simulink model "ckt_notime"  (R2017b)
settings: Solver=VariableStepAuto  StartTime=0.0  StopTime=37790  MaxStep=1e-4  RelTol=1e-3
undefined symbols (not defined in the file or in its folder): sigbuilder_block, Ts_Power
libraries: powerlib x10, re_lib x1, powerlib_meascontrol x1
settings Model: Creator=VSS  LastModifiedBy=VSSDEEP

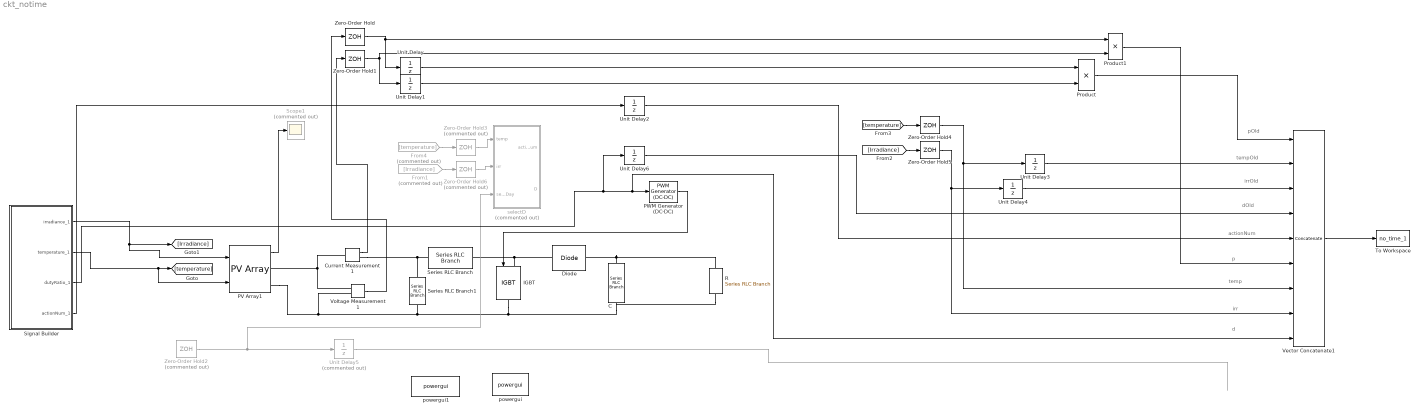
== system ckt_notime ==
  note: d
  note: irr
  note: temp
  note: p
  note: actionNum
  note: dOld
  note: tempOld
  note: irrOld
  note: pOld
  C : powerlib/Elements/Series RLC Branch  LConnTagsString=__new0  RConnTagsString=__new0  BranchType=C  Resistance=5e-3  Inductance=1e-3  SetiL0=off  InitialCurrent=0  Capacitance=330e-6  Setx0=off  InitialVoltage=0  Measurements=None
  Current Measurement1 : powerlib/Measurements/Current Measurement  PhasorSimulation=off  OutputType=Complex  PSBequivalent=0
  Diode : powerlib/Power Electronics/Diode  Ron=0.001  Lon=0  Vf=0.8  IC=0  UseSnubber=off  Rs=500  Cs=250e-9  Measurements=off
  From1 : From  Commented=on  GotoTag=Irradiance
  From4 : From  Commented=on  GotoTag=temperature
  IGBT : powerlib/Power Electronics/IGBT  Ron=0.001  Lon=0  Vf=0  Tf=1e-6  Tt=2e-6  IC=0  Rs=1e5  Cs=inf  Measurements=off
  PV Array1 : re_lib/Solar/PV Array  Npar=1  Nser=1  PlotType=one module @ 25 deg.C & specified irradiances  S_vec="[ 1000  500  100 ]"  Temp_C_vec="[ 45 25  ]"  ModuleName=User-defined  PlotWhenSelected=off  Pm=49.86  Ncell=36  Voc=21.24  Isc=3.05  Vm=18  Im=2.77  beta_Voc_pc=-0.36099  alpha_Isc_pc=0.102  beta_Voc=-0.076674  alpha_Isc=0.003111  IL=3.0546  I0=1.1221e-10  nI=0.95809  Rsh=122.2102  Rs=0.18613  BAL=off  Tc=1e-6  Tfilter=5e-5
  PWM Generator (DC-DC) : powerlib_meascontrol/Pulse & Signal Generators/PWM Generator (DC-DC)  Fsw=25000  Ts=0
  Product : Product
  Product1 : Product
  R : powerlib/Elements/Series RLC Branch  LConnTagsString=__new0  RConnTagsString=__new0  BranchType=R  Resistance=100  Inductance=1e-3  SetiL0=off  InitialCurrent=0  Capacitance=1e-6  Setx0=off  InitialVoltage=0  Measurements=None
  Scope1 : Scope  Commented=on
  Series RLC Branch : powerlib/Elements/Series RLC Branch  LConnTagsString=__new0  RConnTagsString=__new0  BranchType=RL  Resistance=0.001  Inductance=1100e-6  SetiL0=off  InitialCurrent=0  Capacitance=1e-6  Setx0=off  InitialVoltage=0  Measurements=None
  Series RLC Branch1 : powerlib/Elements/Series RLC Branch  LConnTagsString=__new0  RConnTagsString=__new0  BranchType=C  Resistance=1  Inductance=1e-3  SetiL0=off  InitialCurrent=0  Capacitance=1000e-6  Setx0=off  InitialVoltage=0  Measurements=None
  Signal Builder : Subsystem  Tag=STV Subsys  LoadFcn=sigbuilder_block('load');  StartFcn=sigbuilder_block('start');  StopFcn=sigbuilder_block('stop');  ClipboardFcn=sigbuilder_block('clipboard');  mask(Sigbuilder block){tuvar=[0:10]}
      mask help: Simulink:masks:SigbuilderBlock_MD
      mask init:
      | if ~strcmp(get_param(bdroot(gcbh),'SimulationStatus'),'stopped') tuvar = sigbuilder_block('maskInit'); end
      settings: CopyFcn=sigbuilder_block('copy');  DeleteFcn=sigbuilder_block('delete');  ModelCloseFcn=sigbuilder_block('modelClose');  PreSaveFcn=sigbuilder_block('preSave');  PauseFcn=sigbuilder_block('pause');  ContinueFcn=sigbuilder_block('continue');  NameChangeFcn=sigbuilder_block('namechange');  OpenFcn=sigbuilder_block('open',[282.75 137.25 683.25 346.5 ]);  CloseFcn=sigbuilder_block('close');
      mask Display: plot(0, 0, 100, 100,[2, 2, 32, 32, 2], [68, 8, 8, 68, 68],[32, 2], [38, 38], [32, 19, 2],[53, 60, 44], [32, 17, 17, 2],[16, 16, 31, 31]);txt = getActiveGroup(gcbh);text(2, 100, txt,'verticalAlignment', 'top');
  To Workspace : ToWorkspace  VariableName=no_time_1  SampleTime=1
      settings: Save2DSignal=2-D array (concatenate along first dimension)
  Unit Delay{,1..4,6} (6 alike) : UnitDelay
  Unit Delay5 : UnitDelay  Commented=on
  Vector Concatenate1 : Concatenate  NumInputs=9
  Voltage Measurement1 : powerlib/Measurements/Voltage Measurement  PhasorSimulation=off  OutputType=Complex  PSBequivalent=0
  Zero-Order Hold{,1,4..5} (4 alike) : ZeroOrderHold
  Zero-Order Hold2 : ZeroOrderHold  Commented=on
  Zero-Order Hold3 : ZeroOrderHold  Commented=on
  Zero-Order Hold6 : ZeroOrderHold  Commented=on
  powergui : powerlib/powergui  Priority=1  SimulationMode=Continuous  SampleTime=50e-6  frequency=60  Iterations=50  frequencyindice=0  Pbase=100e6  ErrMax=1e-4  UnitsV=kV  UnitsW=MW  buscounter=0  FunctionMessages=off  echomessages=off  EnableUseOfTLC=off  CurrentSourceSwitches=off  DisableSnubberDevices=off  DisableRonSwitches=off  DisableVfSwitches=off  DisplayEquations=off  SolverType=Tustin/Backward Euler (TBE)  Interpol=off  ExternalGateDelay=off  methode=off  Ts=100  x0status=blocks  SPID=on  SwTol=0  HookPort=off  RestoreLinks=warning  ResistiveCurrentMeasurement=off  Frange=[0:2:25000]  Ylog=off  Xlog=on  ShowGrid=off  save=off  variable=ZData  structure=0  ZoomFFT=off  StartTime=0.0  cycles=1  DisplayStyle=1  fundamental=60  FreqAxis=off  MaxFrequency=1000  frequencyindicesteady=1  RmsSteady=1  display=off
  powergui1 : powerlib/powergui  Priority=1  SimulationMode=Continuous  SampleTime=Ts_Power  frequency=60  Iterations=50  frequencyindice=0  Pbase=100e6  ErrMax=1e-4  UnitsV=kV  UnitsW=MW  buscounter=0  FunctionMessages=off  echomessages=off  EnableUseOfTLC=off  CurrentSourceSwitches=off  DisableSnubberDevices=off  DisableRonSwitches=off  DisableVfSwitches=off  DisplayEquations=off  SolverType=Tustin/Backward Euler (TBE)  Interpol=off  ExternalGateDelay=off  methode=off  Ts=100  x0status=blocks  SPID=on  SwTol=0  HookPort=off  RestoreLinks=warning  ResistiveCurrentMeasurement=off  Frange=[0:2:500]  Ylog=off  Xlog=on  ShowGrid=off  save=off  variable=ZData  structure=0  ZoomFFT=on  StartTime=0.0  cycles=1  DisplayStyle=1  fundamental=60  FreqAxis=off  MaxFrequency=1000  frequencyindicesteady=1  RmsSteady=1  display=off
  selectD : MATLAB Function  Commented=on  TreatAsAtomicUnit=on  SystemSampleTime=1
  wires:
  PV Array1/1 -> Scope1/1
  Voltage Measurement1/1 -> Zero-Order Hold/1
  Current Measurement1/1 -> Zero-Order Hold1/1
  Zero-Order Hold4/1 -> Unit Delay3/1, Vector Concatenate1/7
  Zero-Order Hold5/1 -> Unit Delay4/1, Vector Concatenate1/8
  [temperature] -> Zero-Order Hold4/1
  Unit Delay2/1 -> Vector Concatenate1/5
  Unit Delay4/1 -> Vector Concatenate1/3
  Unit Delay/1 -> Product/1
  Unit Delay1/1 -> Product/2
  Unit Delay3/1 -> Vector Concatenate1/2
  [Irradiance] -> Zero-Order Hold5/1
  Zero-Order Hold1/1 -> Product1/2, Unit Delay1/1
  Unit Delay5/1 -> ?
  PWM Generator (DC-DC)/1 -> IGBT/1
  Zero-Order Hold2/1 -> selectD/3(secInDay), Unit Delay5/1
  From1/1 -> Zero-Order Hold6/1
  From4/1 -> Zero-Order Hold3/1
  Zero-Order Hold3/1 -> selectD/1(temp)
  Zero-Order Hold6/1 -> selectD/2(irr)
  Signal Builder/3(dutyRatio_1) -> Unit Delay6/1, PWM Generator (DC-DC)/1, Vector Concatenate1/9
  Product/1 -> Vector Concatenate1/1
  Unit Delay6/1 -> Vector Concatenate1/4
  Product1/1 -> Vector Concatenate1/6
  Zero-Order Hold/1 -> Unit Delay/1, Product1/1
  Vector Concatenate1/1 -> To Workspace/1
  Signal Builder/1(irradiance_1) -> PV Array1/1, [Irradiance]
  Signal Builder/2(temperature_1) -> PV Array1/2, [temperature]
  Signal Builder/4(actionNum_1) -> Unit Delay2/1
  connections:
  Voltage Measurement1/LConn2 -- PV Array1/RConn2 -- Series RLC Branch1/RConn1 -- IGBT/RConn1 -- R/RConn1 -- C/RConn1
  Current Measurement1/LConn1 -- PV Array1/RConn1 -- Voltage Measurement1/LConn1
  Series RLC Branch/RConn1 -- Diode/LConn1 -- IGBT/LConn1
  Series RLC Branch1/LConn1 -- Current Measurement1/RConn1 -- Series RLC Branch/LConn1
  C/LConn1 -- R/LConn1 -- Diode/RConn1

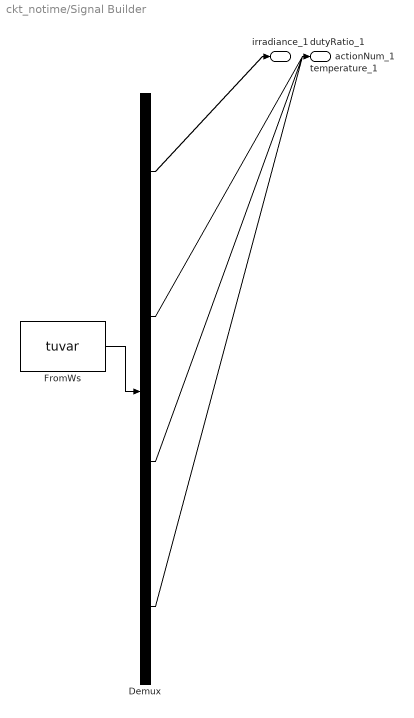
== system ckt_notime/Signal Builder ==
  Demux : Demux  Tag=STV Demux
  FromWs : FromWorkspace  Tag=STV FromWs  VariableName=tuvar  SampleTime=0
      SigBuilderData=|
      | common.afterFinalStr = 'Extrapolate'
      | common.sampleTime = 0
      | dataSet.timeRange = [0 62900]
      | dataSet.name = 'Group 1'
      | sbobj.Groups.Name = 'Group 1'
      | sbobj.Groups.Signals(1).Name = 'irradiance_1'
      | sbobj.Groups.Signals(1).XData = [0 2 3 4 5 6 7 8 9 10 11 12 ... (37790 elements, 1x37790)]
      | sbobj.Groups.Signals(1).YData = [100 100 100 100 100 100 100 100 100 100 100 100 ... (37790 elements, 1x37790)]
      | sbobj.Groups.Signals(2).Name = 'temperature_1'
      | sbobj.Groups.Signals(2).XData = [0 2 3 4 5 6 7 8 9 10 11 12 ... (37790 elements, 1x37790)]
      | sbobj.Groups.Signals(2).YData = [21.5 21.5 21.5 21.5 21.5 21.5 21.5 21.5 21.5 21.5 21.5 21.5 ... (37790 elements, 1x37790)]
      | sbobj.Groups.Signals(3).Name = 'dutyRatio_1'
      | sbobj.Groups.Signals(3).XData = [0 1 2 3 4 5 6 7 8 9 10 11 ... (37792 elements, 1x37792)]
      | sbobj.Groups.Signals(3).YData = [0 0 0.01 0.02 0.03 0.04 0.05 0.06 0.07 0.08 0.09 0.1 ... (37792 elements, 1x37792)]
      | sbobj.Groups.Signals(4).Name = 'actionNum_1'
      | sbobj.Groups.Signals(4).XData = [0 2 3 4 5 6 7 8 9 10 11 12 ... (37790 elements, 1x37790)]
      | sbobj.Groups.Signals(4).YData = [4 4 4 4 4 4 4 4 4 4 4 4 ... (37790 elements, 1x37790)]
      | sbobj.Groups.TimeRange = [0 62900]
  irradiance_1 : Outport  Tag=STV Outport
  temperature_1 : Outport  Tag=STV Outport  Port=2
  dutyRatio_1 : Outport  Tag=STV Outport  Port=3
  actionNum_1 : Outport  Tag=STV Outport  Port=4
  wires:
  FromWs/1 -> Demux/1
  Demux/1 -> irradiance_1/1
  Demux/2 -> temperature_1/1
  Demux/3 -> dutyRatio_1/1
  Demux/4 -> actionNum_1/1

== matlab function ckt_notime/selectD ==
  data: actionNum output; temp input; irr input; D output; secInDay input
function [actionNum, D] = selectD(temp, irr, secInDay)
    %% define some constant
    EPSILON = 1;
    LEVEL_TEMP = 9 ;
    LEVEL_IRR = 9;
    LEVEL_D = 99;
    QTSIZE_STATE = (LEVEL_D+1)*(LEVEL_TEMP+1)*(LEVEL_IRR+1);
    QTSIZE_ACTION = 7;
    TEMP_MAX = 50;
    IRR_MAX = 1300;
    %% load q table  and D
    coder.extrinsic('evalin');
    coder.extrinsic('assignin');
    
    qTable_in = zeros(QTSIZE_STATE, QTSIZE_ACTION);
    if(secInDay<43200)
        qTable_in = evalin('base','qTable_beforeNoon');
    else
        qTable_in = evalin('base','qTable_afterNoon');
    end
    
    oldD = 0;
    oldD = evalin('base','D');
    %% discritalize and normalize
    temp = round( (temp/TEMP_MAX)*LEVEL_TEMP );
    irr = round( (irr/IRR_MAX)*LEVEL_IRR );
    DutyRatio = round(oldD*LEVEL_D);
    %% Epsilon greedy
    if(rand>(1-EPSILON))
        stateNum = ( ( temp*(LEVEL_IRR+1)*(LEVEL_D+1) ) + ( irr*(LEVEL_D+1) ) + DutyRatio)+1 ; % from 0~9999 to 1~ 10000 since MATLAB index starts from 1 
        % [M,I] = max(qTable_in(stateNum,:));
        findMax_original = qTable_in(stateNum,:);
        findMax_randomPos = randperm(QTSIZE_ACTION);
        findMax_shuff = zeros(1, QTSIZE_ACTION);
        for iter = 1:QTSIZE_ACTION
            findMax_shuff(iter) = findMax_original(findMax_randomPos(iter));
        end
        [M,I] = max(findMax_shuff);
        I = findMax_randomPos(I);
    else
        I = randi([1 7],1,1);
    end
    
    actionNum = I;
  
    %% calculate actual D
    D = calculateD(oldD, actionNum);
    assignin('base','D',D);
    
end

function D = calculateD(oldD, actionNum)
    switch actionNum
        case 1
            D = oldD-0.1;
        case 2
            D = oldD-0.05;
        case 3
            D = oldD-0.01;
        case 4
            D = oldD;
        case 5
            D = oldD+0.01;
        case 6
            D = oldD+0.05;
        case 7
            D = oldD+0.1;
        otherwise
            D = oldD; %theorically not possible
    end
    
    if ( D>0.99 )
        D = 0.99; % no short ckt on power mosfet
    end
    if( D<0 )
        D = 0;
    end
    
end
